simulink model "bpsksystem_2023b"  (R2023b)
settings: Solver=ode45  StartTime=0  StopTime=4000  RelTol=1e-3  EnableMultiTasking=on
PreLoadFcn:
  | T =  0.1;         % Symbol period
  | Tc = 0.01;        % Carrier period
  | SNR=15;
  | warning off all
undefined symbols (not defined in the file or in its folder): gcbh, rcfiltgaincompat
libraries: commutil2 x2, commfilt2 x2, commsink2 x1, commchan3 x1, dspfdesign x1, commrandsrc2 x1
settings Model: Creator=Robert Morelos-Zaragoza  LastModifiedBy=14083
settings SolverCC: AlgebraicLoopSolver=TrustRegion
settings DataIOCC: LimitDataPoints=on  SaveFormat=Array  SignalLoggingSaveFormat=ModelDataLogs  ReturnWorkspaceOutputs=off
settings OptimizationCC: ExpressionDepthLimit=2147483647  InitFltsAndDblsToZero=on  LifeSpan=inf
settings DebuggingCC: AlgebraicLoopMsg=none  SaveWithParameterizedLinksMsg=none  UnderspecifiedInitializationDetection=Classic  MergeDetectMultiDrivingBlocksExec=none  SolverPrmCheckMsg=warning  MultiTaskDSMMsg=warning  MultiTaskCondExecSysMsg=none  FcnCallInpInsideContextMsg=warning  UnconnectedInputMsg=warning  UnconnectedOutputMsg=warning  UnconnectedLineMsg=warning  StateNameClashWarn=warning  SFUnexpectedBacktrackingDiag=warning  SFNoUnconditionalDefaultTransitionDiag=warning  SFExecutionAtInitializationDiag=none  ArithmeticOperatorsInVariantConditions=warning
settings HardwareCC: ProdBitPerPointer=32  ProdBitPerSizeT=32  ProdBitPerPtrDiffT=32  ProdLargestAtomicFloat=None  ProdIntDivRoundTo=Undefined  ProdEndianess=Unspecified  ProdWordSize=32  ProdHWDeviceType=32-bit Generic
settings ModelReferenceCC: EnableRefExpFcnMdlSchedulingChecks=on  PropagateSignalLabelsOutOfModel=off
settings SFSimCC: SimUseLocalCustomCode=off  CustomCodeUndefinedFunction=UseInterfaceOnly
settings RTWCC: RTWUseLocalCustomCode=off  DLArmComputeVersion=19.05
settings CodeAppCC: StateflowObjectComments=on
settings GRTTargetCC: TargetFcnLib=ansi_tfl_tmw.mat  TargetLangStandard=C89/C90 (ANSI)  CombineOutputUpdateFcns=off  GRTInterface=on
settings ConfigComp: CovMetricSettings=dw  CovSaveCumulativeToWorkspaceVar=on  CovSaveSingleToWorkspaceVar=on  CovExternalEMLEnable=off

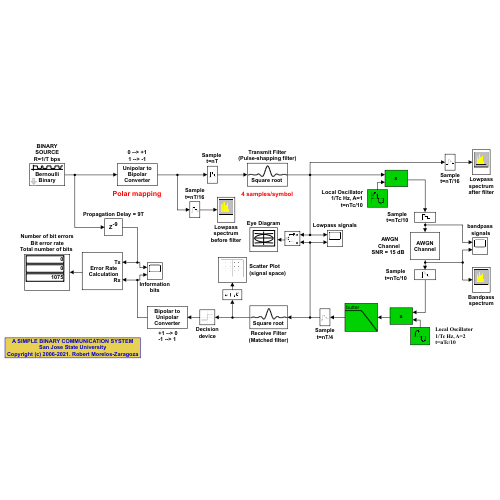
[thumbnail: Simulink's stored preview of the top-level diagram]
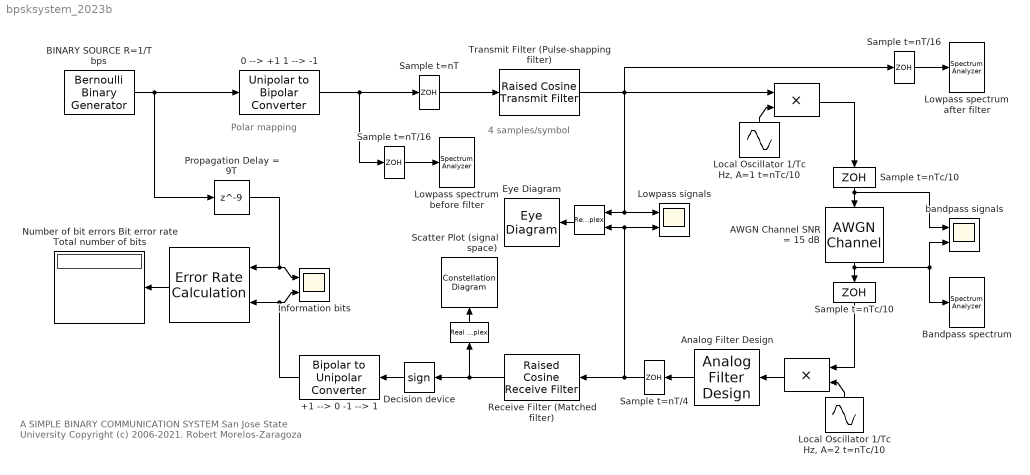
== system bpsksystem_2023b ==
  note: Polar mapping
  note: 4 samples/symbol
  note: A SIMPLE BINARY COMMUNICATION SYSTEM
      | San Jose State University
      | Copyright (c) 2006-2021. Robert Morelos-Zaragoza
  " " : RealImagToComplex
  "   " : Product  InputSameDT=on  SaturateOnIntegerOverflow=on  OutDataTypeStr=Inherit: Same as first input
  "    " : Product  InputSameDT=on  SaturateOnIntegerOverflow=on  OutDataTypeStr=Inherit: Same as first input
  "       " : commsink2/Error Rate Calculation  N=0  st_delay=11  cp_mode=Entire frame  subframe=[]  PMode=Port  WsName=ErrorVec  RsMode2=off  stop=off  numErr=100  maxBits=1e6
  "                 " : RealImagToComplex  Input=Real
  "  Local Oscillator 1/Tc Hz, A=2 t=nTc/10" : Sin  Amplitude=2  Frequency=2*pi/Tc  SampleTime=Tc/10
  "  Sample t=nTc/10  " : ZeroOrderHold  SampleTime=Tc/10
  "  Sample t=nTc/10   " : ZeroOrderHold  SampleTime=Tc/10
  " +1 --> 0 -1 --> 1" : commutil2/Bipolar to Unipolar Converter  M=2  polarity=Negative  dataType=Inherit via internal rule
  0 --> +1 1 --> -1 : commutil2/Unipolar to Bipolar Converter  M=2  polarity=Negative  dataType=Inherit via internal rule
  "AWGN Channel SNR = 15 dB  " : commchan3/AWGN Channel  LegacyMode=on  NoiseMethod="Signal to noise ratio  (SNR)"  noiseMode="Signal to noise ratio  (Eb/No)"  EbNo=SNR  EsNo=15  SNR=10  BitsPerSymbol=1  SignalPower=1  SamplesPerSymbol=1  SymbolPeriod=T/8  VarianceSource=Parameter  Variance=1  RandomStream=Global stream  Seed=67  SimulateUsing=Code generation
  Analog Filter Design : dspfdesign/Analog Filter Design  method=Butterworth  filttype=Lowpass  N=8  Wlo=3*pi/T  Whi=80  Rp=2  Rs=40
  BINARY SOURCE R=1/T bps : commrandsrc2/Bernoulli Binary Generator  P=0.5  seed=61457  Ts=T  frameBased=off  sampPerFrame=1  orient=off  outDataType=double
  Bandpass spectrum : SpectrumAnalyzer  WindowPosition=[4.000000,45.000000,423.000000,261.000000,]  Visible=on  ScopeFrameLocation=window  Method=Welch  SampleRate=1000  PlotAsTwoSidedSpectrum=off  AxesScaling=Manual  FrequencySpan=Start and stop frequencies  Span=500  CenterFrequency=250  StartFrequency=0  StopFrequency=500  FrequencyResolutionMethod=Window length  FFTLengthSource=Property  OverlapPercent=12.5  AveragingMethod=Running  SpectralAverages=30  YLabel=RECEIVED SPECTRUM  YLimits=[-3.9840359254565695935,15.120840798390929649]  DefaultConfigurationName=spbscopes.SpectrumAnalyzerBlockCfg  IsFrequencyInputMode=0  FrequencyVectorPort=0  FrequencyVectorFromPort=0  FrequencyInputRBWPort=0  FrequencyInputRBWFromPort=0  SegLen=1024
  Decision device : Signum
  Eye Diagram : EyeDiagram  Tag=EyeDiagram
  Information bits : Scope  NumInputPorts=2
  "Local Oscillator 1/Tc Hz, A=1 t=nTc/10 " : Sin  Frequency=2*pi/Tc  SampleTime=Tc/10
  Lowpass spectrum after filter : SpectrumAnalyzer  WindowPosition=[437.000000,42.000000,406.000000,262.000000,]  Visible=on  ScopeFrameLocation=window  SpectrumType=Power density  Method=Welch  SampleRate=160  AxesScaling=Manual  FrequencySpan=Start and stop frequencies  Span=160  StartFrequency=-80  StopFrequency=80  FrequencyResolutionMethod=Window length  FFTLengthSource=Property  OverlapPercent=50  AveragingMethod=Running  SpectralAverages=10  SpectrumUnits=dBm/Hz  YLabel=TRANSMITTED BASEBAND SPECTRUM  YLimits=[-30,20]  DefaultConfigurationName=spbscopes.SpectrumAnalyzerBlockCfg  IsFrequencyInputMode=0  FrequencyVectorPort=0  FrequencyVectorFromPort=0  FrequencyInputRBWPort=0  FrequencyInputRBWFromPort=0  SegLen=1024
  Lowpass spectrum before filter : SpectrumAnalyzer  WindowPosition=[437.000000,388.000000,408.000000,264.000000,]  Visible=on  ScopeFrameLocation=window  SpectrumType=Power density  Method=Welch  SampleRate=160  AxesScaling=Manual  FrequencySpan=Start and stop frequencies  Span=160  StartFrequency=-80  StopFrequency=80  FrequencyResolutionMethod=Window length  FFTLengthSource=Property  FFTLength=2048  WindowLength=2048  OverlapPercent=50  AveragingMethod=Running  SpectralAverages=10  SpectrumUnits=dBm/Hz  YLabel=TRANSMITTED BASEBAND SPECTRUM  YLimits=[-20,30]  DefaultConfigurationName=spbscopes.SpectrumAnalyzerBlockCfg  IsFrequencyInputMode=0  FrequencyVectorPort=0  FrequencyVectorFromPort=0  FrequencyInputRBWPort=0  FrequencyInputRBWFromPort=0  SegLen=2048
  Lowpass signals : Scope  NumInputPorts=2
  "Number of bit errors Bit error rate Total number of bits " : Display
  Propagation Delay = 9T : Delay  DelayLength=9  SampleTime=T
  Receive Filter (Matched filter) : commfilt2/Raised Cosine Receive Filter  filtType=Square root  R=1.0  filtSpan=2*(4)  N=4  downFactor=4  downOffset=2  filterGain=(1)*rcfiltgaincompat(gcbh)  InputProcessing=Columns as channels (frame based)  RateOptions=Allow multirate processing  framing=Mute  checkCoeff=off  variableName=rcRxFilt  currentFiltSpan=2*(4)  D=4  inputOffset=0  sampMode=Mute  saveAsFlag=0  rateMode=Downsampling  checkGain=User-specified  launchFVT=off  roundingMode=Floor  overflowMode=off  coeffDataTypeStr=Inherit: Same word length as input  coeffMin=[]  coeffMax=[]  coeffLastDataTypeStr=Inherit: Same word length as input  accumDataTypeStr=Inherit: Same as product output  accumLastDataTypeStr=Inherit: Same as product output  outputDataTypeStr=Inherit: Same as accumulator  outputMin=[]  outputMax=[]  outputLastDataTypeStr=Inherit: Same as accumulator
  "Sample t=nT/16 " : ZeroOrderHold  SampleTime=T/16
  Sample t=nT/16 : ZeroOrderHold  SampleTime=T/16
  Sample t=nT/4 : ZeroOrderHold  SampleTime=T/4
  Sample t=nT : ZeroOrderHold  SampleTime=T
  Scatter Plot (signal space) : ConstellationDiagram  Tag=ScatterPlot  WindowPosition=[846.000000,248.000000,336.000000,341.000000,]  Visible=on  ScopeFrameLocation=window  SymbolsToDisplaySource=Property  SymbolsToDisplay=40  Title=Matched filter output  XLimits=[-1.5 1.5]  YLimits=[-1.5 1.5]  ShowReferenceConstellation=off  ColorFading=on  DefaultConfigurationName=comm.scopes.ConstellationDiagramBlockCfg
  Transmit Filter (Pulse-shapping filter) : commfilt2/Raised Cosine Transmit Filter  filtType=Square root  R=1.0  filtSpan=2*(4)  N=4  filterGain=rcfiltgaincompat(gcbh)  InputProcessing=Columns as channels (frame based)  RateOptions=Allow multirate processing  framing=Mute  checkCoeff=off  variableName=rcTxFilt1  checkGain=Normalized  sampMode=Mute  saveAsFlag=0  currentFiltSpan=2*(4)  D=4  launchFVT=off  roundingMode=Floor  overflowMode=off  coeffDataTypeStr=Inherit: Same word length as input  coeffMin=[]  coeffMax=[]  coeffLastDataTypeStr=Inherit: Same word length as input  outputDataTypeStr=Inherit: Same as accumulator  outputMin=[]  outputMax=[]  outputLastDataTypeStr=Inherit: Same as accumulator
  bandpass signals : Scope  NumInputPorts=2
  wires:
  Propagation Delay = 9T/1 -> "       "/1, Information bits/1
  BINARY SOURCE R=1/T bps/1 -> Propagation Delay = 9T/1, 0 --> +1 1 --> -1/1
  0 --> +1 1 --> -1/1 -> Sample t=nT/16/1, Sample t=nT/1
  "       "/1 -> "Number of bit errors Bit error rate Total number of bits "/1
  Transmit Filter (Pulse-shapping filter)/1 -> "   "/1, "Sample t=nT/16 "/1, " "/1, Lowpass signals/1
  "Local Oscillator 1/Tc Hz, A=1 t=nTc/10 "/1 -> "   "/2
  "   "/1 -> "  Sample t=nTc/10  "/1
  "  Sample t=nTc/10  "/1 -> "AWGN Channel SNR = 15 dB  "/1, bandpass signals/1
  "AWGN Channel SNR = 15 dB  "/1 -> "  Sample t=nTc/10   "/1, bandpass signals/2, Bandpass spectrum/1
  "  Sample t=nTc/10   "/1 -> "    "/1
  "  Local Oscillator 1/Tc Hz, A=2 t=nTc/10"/1 -> "    "/2
  "    "/1 -> Analog Filter Design/1
  Analog Filter Design/1 -> Sample t=nT/4/1
  Sample t=nT/4/1 -> Receive Filter (Matched filter)/1, " "/2, Lowpass signals/2
  Receive Filter (Matched filter)/1 -> Decision device/1, "                 "/1
  Decision device/1 -> " +1 --> 0 -1 --> 1"/1
  " +1 --> 0 -1 --> 1"/1 -> "       "/2, Information bits/2
  " "/1 -> Eye Diagram/1
  "                 "/1 -> Scatter Plot (signal space)/1
  Sample t=nT/16/1 -> Lowpass spectrum before filter/1
  Sample t=nT/1 -> Transmit Filter (Pulse-shapping filter)/1
  "Sample t=nT/16 "/1 -> Lowpass spectrum after filter/1
